simulink model "runHospital"  (Simulink 7.8)
settings: Solver=FixedStepDiscrete  StartTime=0.0  StopTime=inf  FixedStep=60  RelTol=1e-3
settings Model: Creator=mwetter  LastModifiedBy=wbernal  ExtModeAutoUpdateStatusClock=off
settings OptimizationCC: InitFltsAndDblsToZero=on
settings DebuggingCC: SaveWithParameterizedLinksMsg=none  FcnCallInpInsideContextMsg=Use local settings  StrictBusMsg=Warning
settings SFSimCC: SimParseCustomCode=off
settings GRTTargetCC: TargetFcnLib=ansi_tfl_tmw.mat

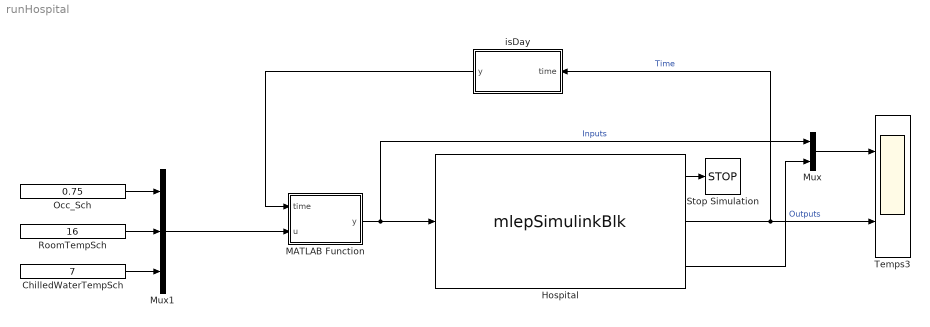
== system runHospital ==
  ChilledWaterTempSch : Constant  Value=7
  Hospital : M-S-Function  FunctionName=mlepSimulinkBlk  Parameters=progname, modelfile, weatherfile, workdir, timeout, port, host, bcvtbdir, deltaT, noutputd  mask(EnergyPlus Cosimulation){progname='C:\\EnergyPlusV8-0-0-mlep\\RunEPlus.bat', modelfile='U:\\Simulink-mlep\\Hospital\\RefBldgHospitalNew2004_Chicago', weatherfile='USA_IL_Chicago-OHare.Intl.AP.725300_TMY3', workdir='U:\\Simulink-mlep\\Hospital', timeout=80000, port=0, host='', bcvtbdir='U:\\Simulink-mlep\\bcvtb', deltaT=60, noutputd=2}
      mask prompts: progname "E+ Executable Path"; modelfile "IDF File (without extension)"; weatherfile "Weather Profile"; workdir "Working Directory"; timeout "Timeout (in milliseconds)"; port "Socket Port (0 = any available)"; host "Socket Host ('' = local host)"; bcvtbdir "BCVTB Directory"; deltaT "Time Step (in seconds)"; noutputd "Number of Real Outputs"
      mask help: This block implements cosimulation with EnergyPlus by allowing Simulink to exchange input and output data with it. Currently, EnergyPlus only supports real data.
      mask Help:
      | This block implements cosimulation with EnergyPlus by allowing Simulink to
      | exchange input and output data with it.
      | 
      | When a simulation starts, EnergyPlus is also started. It will then run in
      | parallel with Simulink. They exchange input and output data via socket
      | communication. When the simulation terminates, EnergyPlus will exit.
      | 
      | Refer to the manuals of MLE+ and/or BCVTB/EnergyPlus for details.
      | 
      | INPUTS:
      | - real: real vector input to EnergyPlus.
      | 
      | OUTPUTS:
      | - flag: status of EnergyPlus (0 if OK, if flag is non-zero, the simulation should stop).
      | - time: current simulation time of EnergyPlus, in seconds.
      | - real: real vector output from EnergyPlus.
      mask Display:
      | disp('E+\nCosimulation');
      | port_label('output', 1, 'flag');
      | port_label('output', 2, 'time');
      | port_label('output', 3, 'real');
      | % port_label('output', 4, 'int');
      | % port_label('output', 5, 'bool');
      | port_label('input', 1, 'real');
      | % port_label('input', 2, 'int');
      | % port_label('input', 3, 'bool');
      | image(imread('Hospital.png'))
  MATLAB Function : MATLAB Function  TreatAsAtomicUnit=on
  Mux : Mux  Inputs=2
  Mux1 : Mux  Inputs=3
  Occ_Sch : Constant  Value=0.75
  RoomTempSch : Constant  Value=16
  Stop Simulation : Stop
  Temps3 : Scope  NumInputPorts=2
      settings: YMin=-5~-5  YMax=5~5
  isDay : Subsystem
  wires:
  Hospital/1 -> Stop Simulation/1
  Hospital/3 -> Mux/2  "Outputs"
  Mux/1 -> Temps3/1
  Mux1/1 -> MATLAB Function/2(u)
  Hospital/2 -> isDay/1(time), Temps3/2  "Time"
  Occ_Sch/1 -> Mux1/1
  RoomTempSch/1 -> Mux1/2
  ChilledWaterTempSch/1 -> Mux1/3
  MATLAB Function/1(y) -> Mux/1, Hospital/1  "Inputs"
  isDay/1(y) -> MATLAB Function/1(time)

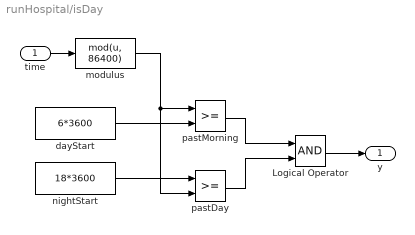
== system runHospital/isDay ==
  time : Inport
  Logical Operator : Logic  AllPortsSameDT=off  OutDataTypeStr=boolean
  dayStart : Constant  Value=6*3600
  modulus : MATLABFcn  MATLABFcn=mod(u, 86400)
  nightStart : Constant  Value=18*3600
  pastDay : RelationalOperator  OutDataTypeStr=boolean
  pastMorning : RelationalOperator  OutDataTypeStr=boolean
  y : Outport
  wires:
  time/1 -> modulus/1
  modulus/1 -> pastMorning/1, pastDay/2
  dayStart/1 -> pastMorning/2
  nightStart/1 -> pastDay/1
  pastMorning/1 -> Logical Operator/1
  pastDay/1 -> Logical Operator/2
  Logical Operator/1 -> y/1

== matlab function MATLAB Function ==
  data: time input double; u input double; y output double
function y = fcn(time, u)
%#codegen

%% BEGIN - CONTROL
K1 = 0.001;
K2 = 0.0001;

% dayTime = mod(time, 86400);
% if (dayTime >= 6*3600) && (dayTime <= 18*3600)
%     if outputs1(2) + outputs2(2) > 9000
%         change = K1*(outputs1(2) + outputs2(2)-9000);
%         chilledWaterTempSch2 = chilledWaterTempSch2 + change;
%     else
%         change = K2*(outputs1(2) + outputs2(2)-9000);
%         chilledWaterTempSch2 = chilledWaterTempSch2 + change;
%     end
%     if chilledWaterTempSch2 < 7
%         chilledWaterTempSch2 = 7;
%     elseif chilledWaterTempSch2 > 10
%         chilledWaterTempSch2 = 10;
%     end
% end
% 
% 
% 
% inputs1 = [airTempSch roomTempSch chilledWaterTempSch1];
 
y = u(1);
